simulink model "WebcamTester5"  (Simulink 7.8)
settings: Solver=FixedStepDiscrete  StartTime=0.0  StopTime=inf  MaxStep=0.2  RelTol=1e-3
settings Model: Creator=gclayton  LastModifiedBy=wildcat
settings DebuggingCC: InheritedTsInSrcMsg=none  FcnCallInpInsideContextMsg=Use local settings  StrictBusMsg=Warning
settings SFSimCC: SimParseCustomCode=off
settings RTWCC: SystemTargetFile=rlnx.tlc  GenCodeOnly=on  TemplateMakefile=rlnx_ubuntu.tmf  Description=Linux Real-Time Target  ProcessScript=rlnx_make_rtw_hook
settings RTWCC: CustomInclude=|
  | /usr/local/include/opencv/
  | /usr/local/include/
  | /usr/local/lib/
settings CodeAppCC: GenerateComments=off  SimulinkBlockComments=off
settings STFCustomTargetCC: ModelReferenceCompliant=off  MatFileLogging=on  SystemTargetFile=rlnx.tlc
settings GRTTargetCC: ModelReferenceCompliant=off  ParMdlRefBuildCompliant=off  CompOptLevelCompliant=off  ConcurrentExecutionCompliant=off
settings CustomProperty: DataType=string  Value=-lm -ldl /usr/local/lib/libopencv_highgui.so.2.4 /usr/local/lib/libopencv_core.so.2.4 /usr/local/lib/libopencv_calib3d.so.2.4 /usr/local/lib/libopencv_contrib.so.2.4 /usr/local/lib/libopencv_features2d.so.2.4 /usr/local/lib/libopencv_flann.so.2.4 /usr/local/lib/libopencv_gpu.so.2.4 /usr/local/lib/libopencv_imgproc.so.2.4 /usr/local/lib/libopencv_legacy.so.2.4 /usr/local/lib/libopencv_ml.so.2.4 /usr/local/lib/libopencv_nonfree.so.2.4 /usr/local/lib/libopencv_objdetect.so.2.4 /usr/local/lib/libopencv_photo.so.2.4 /usr/local/lib/libopencv_stitching.so.2.4 /usr/local/lib/libopencv_ts.so.2.4 /usr/local/lib/libopencv_video.so.2.4 /usr/local/lib/libopencv_videostab.so.2.4
settings EnumStrPairs: String=PC

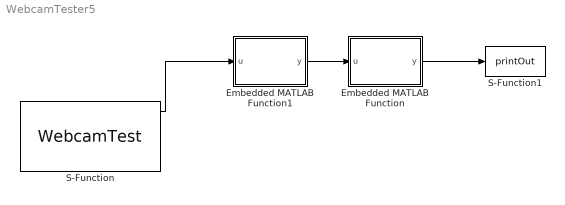
== system WebcamTester5 ==
  Embedded MATLAB Function : MATLAB Function  TreatAsAtomicUnit=on
  Embedded MATLAB Function1 : MATLAB Function  TreatAsAtomicUnit=on
  S-Function : S-Function  FunctionName=WebcamTest  EnableBusSupport=off
  S-Function1 : S-Function  FunctionName=printOut  EnableBusSupport=off
  wires:
  S-Function/1 -> Embedded MATLAB Function1/1(u)
  Embedded MATLAB Function/1(y) -> S-Function1/1
  Embedded MATLAB Function1/1(y) -> Embedded MATLAB Function/1(u)

== matlab function Embedded MATLAB Function1 ==
  data: u input double; y output double
function y = fcn(u)

y = uint32(u);

== matlab function Embedded MATLAB Function ==
  data: u input double; y output double
function y = fcn(u)

y = u(100,100);
